simulink model "system_model"  (R2021a)
settings: Solver=VariableStepAuto  StartTime=0.0  StopTime=1000  RelTol=1e-3
values from neighbouring files (symbols this model uses):
  den = sys.Denominator    [backup.m]    (also in tf_estimate.m)
  kp = 1/mag(1,1,min(k))    [backup.m]    (also in tf_estimate.m = 1/mag(k))
  num = sys.Numerator    [backup.m]    (also in tf_estimate.m)
  ti = Ni*1/wc    [backup.m]    (also in tf_estimate.m)
undefined symbols (not defined in the file or in its folder): sat_limit
settings Model: Creator=leouh  LastModifiedBy=leouh

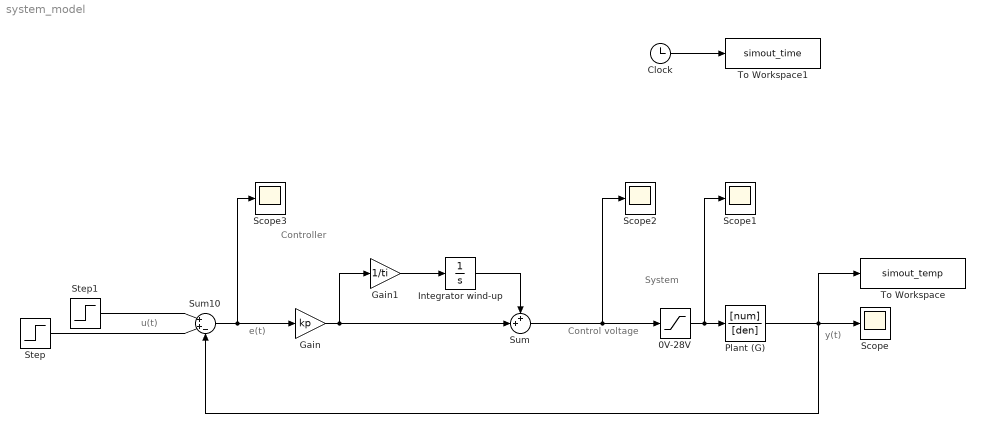
== system system_model ==
  note: y(t)
  note: u(t)
  note: e(t)
  note: System
  note: Controller
  note: Control voltage
  0V-28V : Saturate  UpperLimit=28  LowerLimit=0
  Clock : Clock
  Gain : Gain  Gain=kp
  Gain1 : Gain  Gain=1/ti
  Integrator wind-up : Integrator  LimitOutput=on  UpperSaturationLimit=sat_limit  LowerSaturationLimit=0
  Plant (G) : TransferFcn  Numerator=[num]  Denominator=[den]
  Scope{,1..3} (4 alike) : Scope
  Step : Step  After=175  SampleTime=0
  Step1 : Step  Time=600  After=-10  SampleTime=0
  Sum : Sum  Inputs=++|
  Sum10 : Sum  Inputs=|++-
  To Workspace : ToWorkspace  VariableName=simout_temp  SaveFormat=Timeseries  SampleTime=-1
  To Workspace1 : ToWorkspace  VariableName=simout_time  SaveFormat=Timeseries  SampleTime=-1
  wires:
  Sum10/1 -> Scope3/1, Gain/1
  Plant (G)/1 -> To Workspace/1, Sum10/3, Scope/1
  0V-28V/1 -> Scope1/1, Plant (G)/1
  Gain1/1 -> Integrator wind-up/1
  Gain/1 -> Sum/2, Gain1/1
  Step/1 -> Sum10/2
  Step1/1 -> Sum10/1
  Integrator wind-up/1 -> Sum/1
  Sum/1 -> Scope2/1, 0V-28V/1
  Clock/1 -> To Workspace1/1
